simulink model "soru1e"  (R2019a)
settings: Solver=VariableStepAuto  StartTime=0.0  StopTime=30  RelTol=1e-3
settings Model: Creator=handeyildirim  LastModifiedBy=handeyildirim

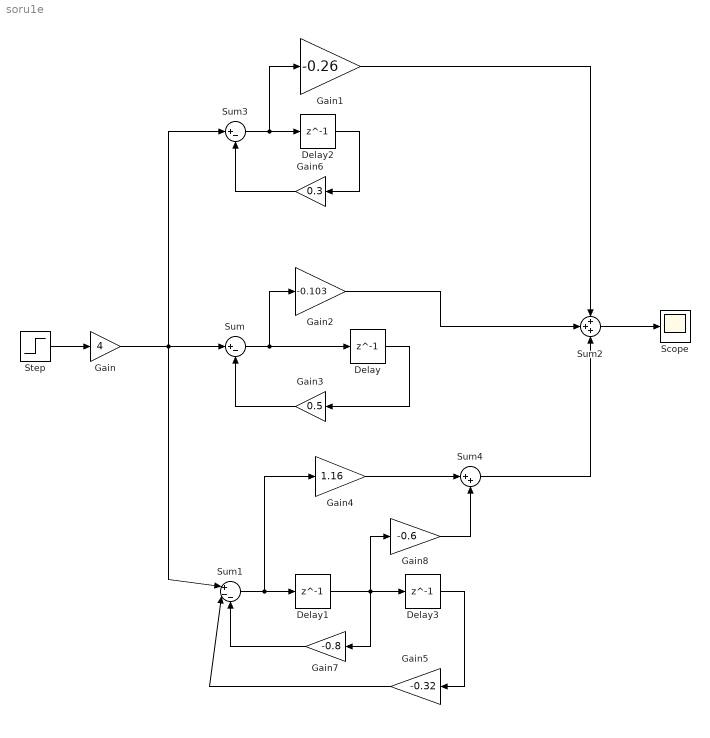
== system soru1e ==
  Delay{,1..3} (4 alike) : Delay  DelayLength=1
  Gain : Gain  Gain=4
  Gain1 : Gain  Gain=-0.26
  Gain2 : Gain  Gain=-0.103
  Gain3 : Gain  Gain=0.5
  Gain4 : Gain  Gain=1.16
  Gain5 : Gain  Gain=-0.32
  Gain6 : Gain  Gain=0.3
  Gain7 : Gain  Gain=-0.8
  Gain8 : Gain  Gain=-0.6
  Scope : Scope
  Step : Step  SampleTime=1
  Sum : Sum  Inputs=|+-
  Sum1 : Sum  Inputs=|+--
  Sum2 : Sum  Inputs=+++
  Sum3 : Sum  Inputs=|+-
  Sum4 : Sum  Inputs=|++
  wires:
  Step/1 -> Gain/1
  Sum/1 -> Gain2/1, Delay/1
  Gain3/1 -> Sum/2
  Delay/1 -> Gain3/1
  Gain2/1 -> Sum2/2
  Sum1/1 -> Gain4/1, Delay1/1
  Gain5/1 -> Sum1/2
  Sum2/1 -> Scope/1
  Gain/1 -> Sum3/1, Sum1/1, Sum/1
  Delay2/1 -> Gain6/1
  Gain1/1 -> Sum2/1
  Sum3/1 -> Gain1/1, Delay2/1
  Gain6/1 -> Sum3/2
  Delay1/1 -> Gain7/1, Delay3/1, Gain8/1
  Delay3/1 -> Gain5/1
  Gain7/1 -> Sum1/3
  Gain4/1 -> Sum4/1
  Gain8/1 -> Sum4/2
  Sum4/1 -> Sum2/3
